simulink model "bp5b_model"  (R2022a)
settings: Solver=ode45  StartTime=0.0  StopTime=10.0  RelTol=1e-10
PreLoadFcn:
  | alpha=[0.5,0.1,1,0.5]; x0=[1,0.3,0.5,1];
  |    ww=[1e-6, 1e6]; N=33;
undefined symbols (not defined in the file): G
libraries: cstblocks x4
settings Model: Creator=xuedi  LastModifiedBy=xuedi
settings DataIOCC: SaveFormat=Array  ReturnWorkspaceOutputs=off

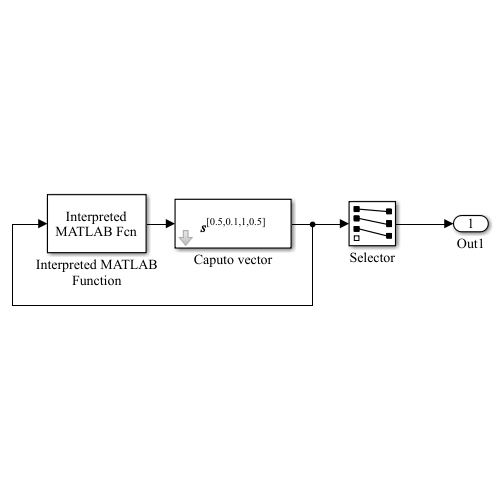
[thumbnail: Simulink's stored preview of the top-level diagram]
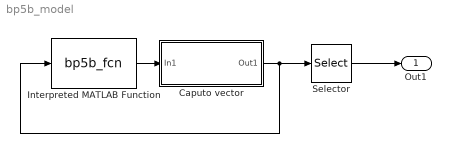
== system bp5b_model ==
  Caputo vector : Subsystem  mask{gam=alpha, ww=ww, N=N, M=4, x0=x0}
      mask prompts: gam "Derivative order gamma"; ww "Frequency range [wb,wh]"; N "Approximation order N"; M "Dimension M"; x0 "Initial condition x0"
      mask init:
      | wb=ww(1); wh=ww(2); stri=[];
      |    if length(gam)==1, gam=gam*ones(M,1); end
      |    for i=1:M
      |        G(i,1)=ousta_fod(1-gam(i),N,wb,wh); stri=[stri,num2str(gam(i)),','];
      |    end
      |    str=['{\bf{\its}}^{[' stri(1:end-1) ']}'];
      |    svec2sl(gam);
      mask Display: disp(str,'texmode','on')
  Interpreted MATLAB Function : MATLABFcn  MATLABFcn=bp5b_fcn  OutputDimensions=4  Output1D=off
  Selector : Selector  InputPortWidth=4  IndexOptions=Index vector (dialog)  Indices=[1 2 3]  OutputSizes=1
  Out1 : Outport
  wires:
  Interpreted MATLAB Function/1 -> Caputo vector/1(In1)
  Caputo vector/1(Out1) -> Selector/1, Interpreted MATLAB Function/1
  Selector/1 -> Out1/1

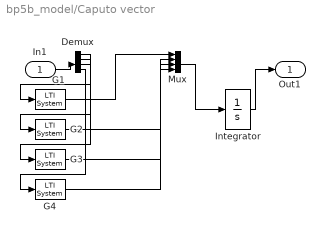
== system bp5b_model/Caputo vector ==
  In1 : Inport
  Demux : Demux
  G1 : cstblocks/LTI System  sys=G(1)  IC=[]
  G2 : cstblocks/LTI System  sys=G(2)  IC=[]
  G3 : cstblocks/LTI System  sys=G(3)  IC=[]
  G4 : cstblocks/LTI System  sys=G(4)  IC=[]
  Integrator : Integrator  InitialCondition=x0
  Mux : Mux
  Out1 : Outport
  wires:
  Demux/1 -> G1/1
  G1/1 -> Mux/1
  Demux/2 -> G2/1
  G2/1 -> Mux/2
  Demux/3 -> G3/1
  G3/1 -> Mux/3
  Demux/4 -> G4/1
  G4/1 -> Mux/4
  Integrator/1 -> Out1/1
  Mux/1 -> Integrator/1
  In1/1 -> Demux/1
